simulink model "SaturateDemo"  (Simulink 6.3)
settings: Solver=FixedStepDiscrete  StartTime=0.0  StopTime=10.0  FixedStep=1  RelTol=1e-3
InitFcn:
  | %% DSPBuilder Start
  | alt_dspbuilder_update_model(bdroot)
  | %% DSPBuilder End
libraries: allblocks_alteradspbuilder2 x7
settings Model: LastModifiedBy=delphick

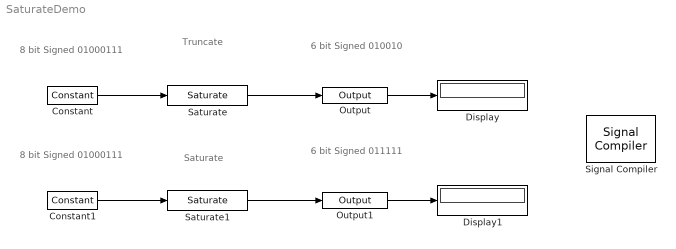
== system SaturateDemo ==
  note: 8 bit Signed
      | 01000111
  note: 6 bit Signed
      | 010010
  note: 8 bit Signed
      | 01000111
  note: 6 bit Signed
      | 011111
  note: Truncate
  note: Saturate
  Constant : allblocks_alteradspbuilder2/Constant  mask_cst=71  BusType=Signed Integer  bwl=8  bwr=0  SpecifyClock=off
  Constant1 : allblocks_alteradspbuilder2/Constant  mask_cst=71  BusType=Signed Integer  bwl=8  bwr=0  SpecifyClock=off
  Display : Display
  Display1 : Display
  Output : allblocks_alteradspbuilder2/Output  iofile=C:\workspace_clean\Documentation\DesignExamples\Tutorials\UnitBlocks\IOBus\Saturate\tb_SaturateDemo\SaturateDemo_Output.capture  BusType=Signed Integer  bwl=6  bwr=0  PORTTYPE=Output
  Output1 : allblocks_alteradspbuilder2/Output  iofile=C:\workspace_clean\Documentation\DesignExamples\Tutorials\UnitBlocks\IOBus\Saturate\tb_SaturateDemo\SaturateDemo_Output1.capture  BusType=Signed Integer  bwl=6  bwr=0  PORTTYPE=Output
  Saturate : allblocks_alteradspbuilder2/Saturate  BusType=Signed Integer  bwl=8  bwr=0  bitsToRemove=2  satMode=Truncate MSB  UpperLimit=0  LowerLimit=0  pipeline=off
  Saturate1 : allblocks_alteradspbuilder2/Saturate  BusType=Signed Integer  bwl=8  bwr=0  bitsToRemove=2  satMode=Saturate  UpperLimit=0  LowerLimit=0  pipeline=off
  Signal Compiler : allblocks_alteradspbuilder2/Signal Compiler  DeviceFamily=Stratix IV  DeviceName=AUTO  EnableSignalTap=off  SignalTapDepth=128  UseBoardBlock=off  StpUseDefaultClock=on  StpClock=clock
  wires:
  Constant/1 -> Saturate/1
  Saturate/1 -> Output/1
  Output/1 -> Display/1
  Constant1/1 -> Saturate1/1
  Saturate1/1 -> Output1/1
  Output1/1 -> Display1/1
